simulink model "model"  (R2019b)
settings: Solver=VariableStepAuto  StartTime=0.0  StopTime=80.0  RelTol=1e-3
values from neighbouring files (symbols this model uses):
  c = 0.00035    [constants.m]
  d = 0.023    [constants.m]
  g = 9.80665    [constants.m]
  J = 0.0090    (= 0.009)    [constants.m]
  L = 0.495    [constants.m]
  m = 0.43    [constants.m]
libraries: simulink_extras x2, fuzblock x1
settings Model: SimulationMode=accelerator  Creator=josepdecidrodriguez  LastModifiedBy=gonzalo
settings SolverCC: ZeroCrossControl=DisableAll
settings OptimizationCC: BooleanDataType=off

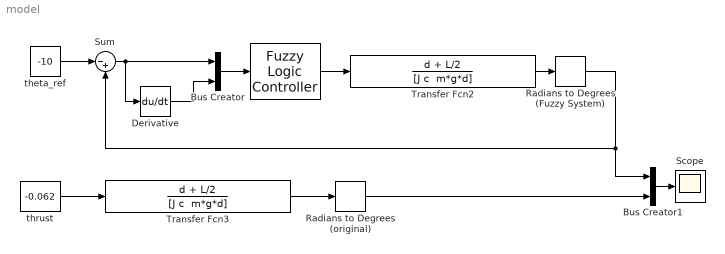
== system model ==
  " " : fuzblock/Fuzzy Logic  Controller  FIS=fismat  OutputSampleNumber=101  DataType=double  FuzzifiedInputs=off  RuleFiringStrengths=off  RuleOutputs=off  AggregatedOutputs=off  SimulateUsing=Interpreted execution  OutOfRangeInputValueMessage=warning  NoRuleFiredMessage=warning  EmptyOutputFuzzySetMessage=warning
  Bus Creator : BusCreator  Inputs=2
  Bus Creator1 : BusCreator  Inputs=2
  "Derivative " : Derivative
  Radians to Degrees (Fuzzy System) : simulink_extras/Transformations/Radians to Degrees
  Radians to Degrees (original) : simulink_extras/Transformations/Radians to Degrees
  Scope : Scope
  Sum : Sum  Inputs=|-+
  Transfer Fcn2 : TransferFcn  Numerator=d + L/2  Denominator="[J c  m*g*d]"
  Transfer Fcn3 : TransferFcn  Numerator=d + L/2  Denominator="[J c  m*g*d]"
  theta_ref : Constant  Value=-10
  thrust : Constant  Value=-0.062
  wires:
  theta_ref/1 -> Sum/1
  Sum/1 -> Bus Creator/1, "Derivative "/1
  "Derivative "/1 -> Bus Creator/2
  Bus Creator/1 -> " "/1
  " "/1 -> Transfer Fcn2/1
  Transfer Fcn2/1 -> Radians to Degrees (Fuzzy System)/1
  Radians to Degrees (Fuzzy System)/1 -> Sum/2, Bus Creator1/1
  Bus Creator1/1 -> Scope/1
  Radians to Degrees (original)/1 -> Bus Creator1/2
  thrust/1 -> Transfer Fcn3/1
  Transfer Fcn3/1 -> Radians to Degrees (original)/1
